simulink model "exam3_sim_2"  (R2023a)
settings: Solver=FixedStepAuto  StartTime=0.0  StopTime=4  FixedStep=Tvz  RelTol=1e-3
values from neighbouring files (symbols this model uses):
  B = 0.0024    [I-PD_pole-placement.mat]    (also in PIV.mat; dobre_pid.mat; exam3.m; exam3_2.m)
  J_m = 0.005    [I-PD_pole-placement.mat]    (also in PIV.mat; dobre_pid.mat; exam3.m; exam3_2.m)
  k_d = 0.2847    [I-PD_pole-placement.mat]    (also in dobre_pid.mat = 0.712758975447; exam3_2.m)
  k_i = 67.5    [I-PD_pole-placement.mat]    (also in PIV.mat = 2.36572; dobre_pid.mat = 0.0660293176822; exam3.m = 4.828; exam3_2.m)
  k_p = 7.6815    [I-PD_pole-placement.mat]    (also in PIV.mat = 5.79950289975; dobre_pid.mat = 8.78704740486; exam3.m = 8.2850041425; exam3_2.m)
  M_n = 6.4    [I-PD_pole-placement.mat]    (also in PIV.mat; dobre_pid.mat; exam3.m; exam3_2.m)
  Nel = 10000    [I-PD_pole-placement.mat]    (also in PIV.mat; dobre_pid.mat; exam3.m; exam3_2.m)
  T_n = 0.015    [I-PD_pole-placement.mat]    (also in PIV.mat; dobre_pid.mat; exam3.m; exam3_2.m)
  Tvz = 0.004    [I-PD_pole-placement.mat]    (also in PIV.mat; dobre_pid.mat; exam3.m; exam3_2.m)
undefined symbols (not defined in the file or in its folder): DiscIntNeverNeededParam
libraries: simulink x2, SignalEditorBlockLib x1
settings Model: Creator=laptop  LastModifiedBy=laptop

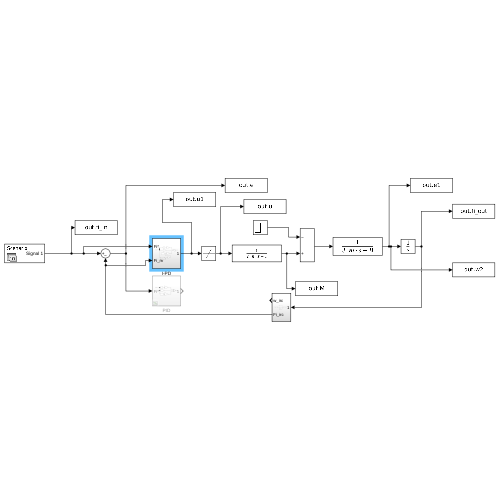
[thumbnail: Simulink's stored preview of the top-level diagram]
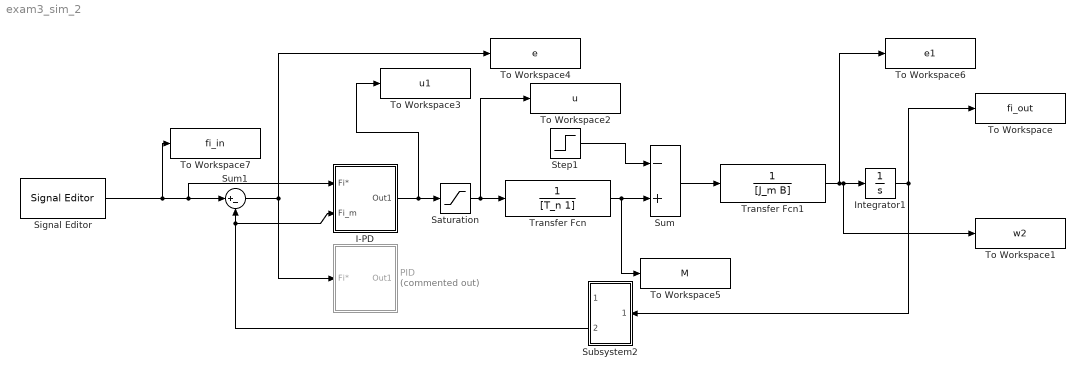
== system exam3_sim_2 ==
  I-PD : Subsystem
  Integrator1 : Integrator
  PID : Subsystem  Commented=on
  Saturation : Saturate  UpperLimit=M_n*0.75  LowerLimit=-M_n*0.75
  Signal Editor : SignalEditorBlockLib/Signal Editor  FileName=signalmat.mat  ActiveScenario=Scenario  ActiveSignal=Signal 1  IsBus=off  OutputBusObjectStr=Bus: BusObject  SampleTime=0  Interpolate=off  ZeroCross=off  OutputAfterFinalValue=Holding final value  Unit=inherit  PreserveSignalName=on  ApplySigPropsToAllScenarios=on
  Step1 : Step  After=M_n*0.1  SampleTime=0
  Subsystem2 : Subsystem
  Sum : Sum  Inputs=-+
  Sum1 : Sum  Inputs=|+-
  To Workspace : ToWorkspace  VariableName=fi_out  SaveFormat=Timeseries  SampleTime=-1
  To Workspace1 : ToWorkspace  VariableName=w2  SaveFormat=Timeseries  SampleTime=-1
  To Workspace2 : ToWorkspace  VariableName=u  SaveFormat=Timeseries  SampleTime=-1
  To Workspace3 : ToWorkspace  VariableName=u1  SaveFormat=Timeseries  SampleTime=-1
  To Workspace4 : ToWorkspace  VariableName=e  SaveFormat=Timeseries  SampleTime=-1
  To Workspace5 : ToWorkspace  VariableName=M  SaveFormat=Timeseries  SampleTime=-1
  To Workspace6 : ToWorkspace  VariableName=e1  SaveFormat=Timeseries  SampleTime=-1
  To Workspace7 : ToWorkspace  VariableName=fi_in  SaveFormat=Timeseries  SampleTime=-1
  Transfer Fcn : TransferFcn  Denominator=[T_n 1]
  Transfer Fcn1 : TransferFcn  Denominator=[J_m B]
  wires:
  Transfer Fcn/1 -> To Workspace5/1, Sum/2
  Saturation/1 -> Transfer Fcn/1, To Workspace2/1
  Sum/1 -> Transfer Fcn1/1
  Transfer Fcn1/1 -> To Workspace6/1, To Workspace1/1, Integrator1/1
  Step1/1 -> Sum/1
  Signal Editor/1 -> To Workspace7/1, I-PD/1(Fi*), Sum1/1
  Integrator1/1 -> Subsystem2/1(In1), To Workspace/1
  Subsystem2/2(Fi_irc) -> I-PD/2(Fi_m), Sum1/2
  I-PD/1(Out1) -> To Workspace3/1, Saturation/1
  Sum1/1 -> To Workspace4/1, PID/1(Fi*)

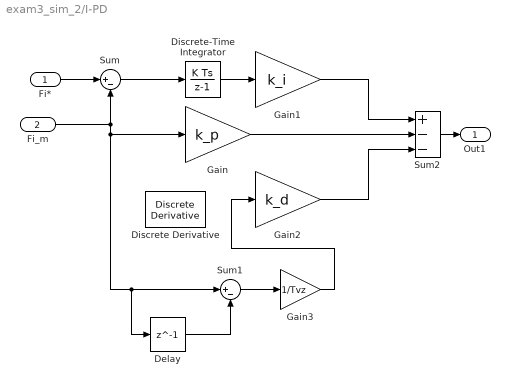
== system exam3_sim_2/I-PD ==
  Fi* : Inport
  Fi_m : Inport  Port=2
  Delay : Delay  DelayLength=1
  Discrete Derivative : simulink/Discrete/Discrete Derivative  gainval=1.0  ICPrevScaledInput=0.0  OutMin=[]  OutMax=[]  OutDataType=fixdt(1, 16)  OutScaling=2^-10  DoSatur=off
  Discrete-Time Integrator : DiscreteIntegrator  SampleTime=Tvz  ICPrevOutput=DiscIntNeverNeededParam  ICPrevScaledInput=DiscIntNeverNeededParam
  Gain : Gain  Gain=k_p
  Gain1 : Gain  Gain=k_i
  Gain2 : Gain  Gain=k_d
  Gain3 : Gain  Gain=1/Tvz
  Sum : Sum  Inputs=|+-
  Sum1 : Sum  Inputs=|+-
  Sum2 : Sum  Inputs=+--
  Out1 : Outport
  wires:
  Discrete-Time Integrator/1 -> Gain1/1
  Gain2/1 -> Sum2/3
  Sum1/1 -> Gain3/1
  Gain/1 -> Sum2/2
  Sum2/1 -> Out1/1
  Gain1/1 -> Sum2/1
  Fi*/1 -> Sum/1
  Sum/1 -> Discrete-Time Integrator/1
  Fi_m/1 -> Delay/1, Sum1/1, Gain/1, Sum/2
  Delay/1 -> Sum1/2
  Gain3/1 -> Gain2/1

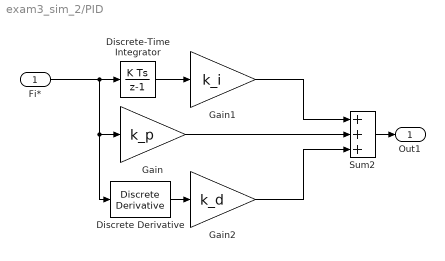
== system exam3_sim_2/PID ==
  Fi* : Inport
  Discrete Derivative : simulink/Discrete/Discrete Derivative  gainval=1.0  ICPrevScaledInput=0.0  OutMin=[]  OutMax=[]  OutDataType=fixdt(1, 16)  OutScaling=2^-10  DoSatur=off
  Discrete-Time Integrator : DiscreteIntegrator  SampleTime=Tvz  ICPrevOutput=DiscIntNeverNeededParam  ICPrevScaledInput=DiscIntNeverNeededParam
  Gain : Gain  Gain=k_p
  Gain1 : Gain  Gain=k_i
  Gain2 : Gain  Gain=k_d
  Sum2 : Sum  Inputs=+++
  Out1 : Outport
  wires:
  Discrete-Time Integrator/1 -> Gain1/1
  Gain2/1 -> Sum2/3
  Discrete Derivative/1 -> Gain2/1
  Gain/1 -> Sum2/2
  Sum2/1 -> Out1/1
  Gain1/1 -> Sum2/1
  Fi*/1 -> Discrete Derivative/1, Gain/1, Discrete-Time Integrator/1

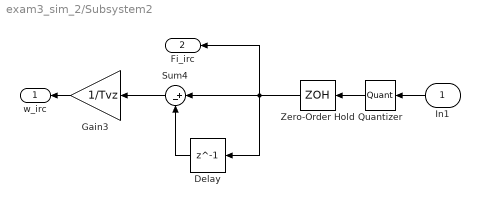
== system exam3_sim_2/Subsystem2 ==
  In1 : Inport
  Delay : Delay  DelayLength=1
  Gain3 : Gain  Gain=1/Tvz
  Quantizer : Quantizer  QuantizationInterval=2*pi/Nel
  Sum4 : Sum  Inputs=|+-
  Zero-Order Hold : ZeroOrderHold  SampleTime=Tvz
  w_irc : Outport
  Fi_irc : Outport  Port=2
  wires:
  Sum4/1 -> Gain3/1
  Delay/1 -> Sum4/2
  Zero-Order Hold/1 -> Delay/1, Sum4/1, Fi_irc/1
  In1/1 -> Quantizer/1
  Quantizer/1 -> Zero-Order Hold/1
  Gain3/1 -> w_irc/1
